simulink model "DLH_BDK_PD_momen_PP_r2014b"  (R2014b)
settings: Solver=ode3  SolverMode=SingleTasking  StartTime=0.0  StopTime=10  FixedStep=0.001  RelTol=1e-3
undefined symbols (not defined in the file): ADAMS_cwd, ADAMS_exec, ADAMS_host, ADAMS_init, ADAMS_inputs, ADAMS_outputs, ADAMS_prefix, ADAMS_static, ADAMS_sysdir
libraries: simulink x1
settings Model: CovMetricSettings=dwe  CovHtmlReporting=off  covSaveCumulativeToWorkspaceVar=off  CovSaveSingleToWorkspaceVar=off  CovExternalEMLEnable=on  CovSFcnEnable=on  Creator=MTA  LastModifiedBy=Administrator
settings DataIOCC: LimitDataPoints=off  SaveFormat=StructureWithTime
settings DebuggingCC: SolverPrmCheckMsg=none  FrameProcessingCompatibilityMsg=error  SFUnexpectedBacktrackingDiag=error  SFNoUnconditionalDefaultTransitionDiag=error
settings HardwareCC: ProdBitPerPointer=64  ProdLargestAtomicFloat=Float  ProdIntDivRoundTo=Zero  ProdEndianess=LittleEndian  ProdHWDeviceType=Specified
settings ModelReferenceCC: PropagateSignalLabelsOutOfModel=on
settings GRTTargetCC: TargetLangStandard=C99 (ISO)  GeneratePreprocessorConditionals=Use local settings

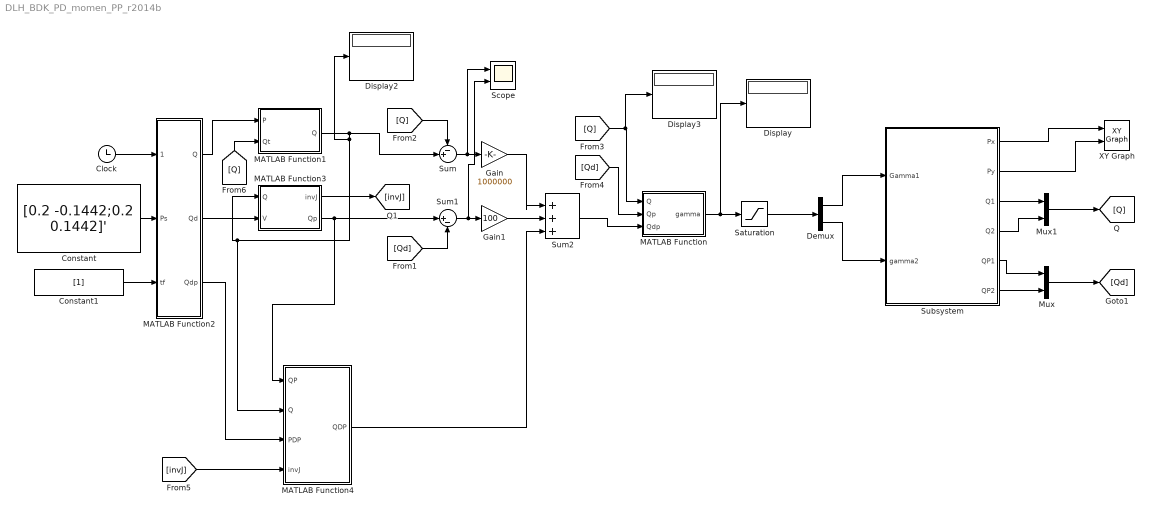
== system DLH_BDK_PD_momen_PP_r2014b ==
  Clock : Clock
  Constant : Constant  Value="[0.2  -0.1442;0.2 0.1442]'"
  Constant1 : Constant  Value=[1]
  Demux : Demux  Outputs=2
  Display : Display
  Display2 : Display
  Display3 : Display
  Gain : Gain  Gain=1000000
  Gain1 : Gain  Gain=100
  MATLAB Function : MATLAB Function  TreatAsAtomicUnit=on
      settings: PermitHierarchicalResolution=ParametersOnly
  MATLAB Function1 : MATLAB Function  TreatAsAtomicUnit=on
      settings: PermitHierarchicalResolution=ParametersOnly
  MATLAB Function2 : MATLAB Function  TreatAsAtomicUnit=on
      settings: PermitHierarchicalResolution=ParametersOnly
  MATLAB Function3 : MATLAB Function  TreatAsAtomicUnit=on
      settings: PermitHierarchicalResolution=ParametersOnly
  MATLAB Function4 : MATLAB Function  TreatAsAtomicUnit=on
      settings: PermitHierarchicalResolution=ParametersOnly
  Mux : Mux  Inputs=2
  Mux1 : Mux  Inputs=2
  Saturation : Saturate  UpperLimit=[5;5]  LowerLimit=[-5;-5]
  Scope : Scope  NumInputPorts=2
      settings: TimeRange=auto  MaxDataPoints=5000  SaveToWorkspace=off  SaveName=ScopeData  YMin=-469.58587~-5  YMax=523.49918~5  SampleTime=-1
  Subsystem : Subsystem
  Sum : Sum  Inputs=-+|
  Sum1 : Sum  Inputs=|+-
  Sum2 : Sum  Inputs=|+++
  XY Graph : simulink/Sinks/XY Graph  xmin=-1  xmax=1  ymin=-1  ymax=1  st=-1
  wires:
  Constant/1 -> MATLAB Function2/2(Ps)
  Constant1/1 -> MATLAB Function2/3(tf)
  Clock/1 -> MATLAB Function2/1(time)
  Sum/1 -> Scope/1, Gain/1
  Gain/1 -> Sum2/1
  Gain1/1 -> Sum2/2
  Sum1/1 -> Scope/2, Gain1/1
  Sum2/1 -> MATLAB Function/3(Qdp)
  Subsystem/2("Py ") -> XY Graph/2
  Subsystem/1("Px ") -> XY Graph/1
  Mux1/1 -> [Q]
  Mux/1 -> [Qd]
  Demux/2 -> Subsystem/2(gamma2)
  Subsystem/6(QP2) -> Mux/2
  Demux/1 -> Subsystem/1(Gamma1)
  Subsystem/4("Q2 ") -> Mux1/2
  Subsystem/3("Q1 ") -> Mux1/1
  Subsystem/5(QP1) -> Mux/1
  Saturation/1 -> Demux/1
  [Q] -> Sum/1
  [Qd] -> Sum1/2
  [Q] -> Display3/1, MATLAB Function/1(Q)
  MATLAB Function/1(gamma) -> Display/1, Saturation/1
  [Qd] -> MATLAB Function/2(Qp)
  MATLAB Function2/1(Q) -> MATLAB Function1/1(P)
  MATLAB Function1/1(Q) -> MATLAB Function4/2(Q), MATLAB Function3/1(Q), Display2/1, Sum/2
  MATLAB Function3/2(Qp) -> MATLAB Function4/1(QP), Sum1/1
  MATLAB Function2/2(Qd) -> MATLAB Function3/2(V)
  MATLAB Function2/3(Qdp) -> MATLAB Function4/3(PDP)
  MATLAB Function3/1(invJ) -> [invJ]
  [invJ] -> MATLAB Function4/4(invJ)
  MATLAB Function4/1(QDP) -> Sum2/3
  [Q] -> MATLAB Function1/2(Qt)

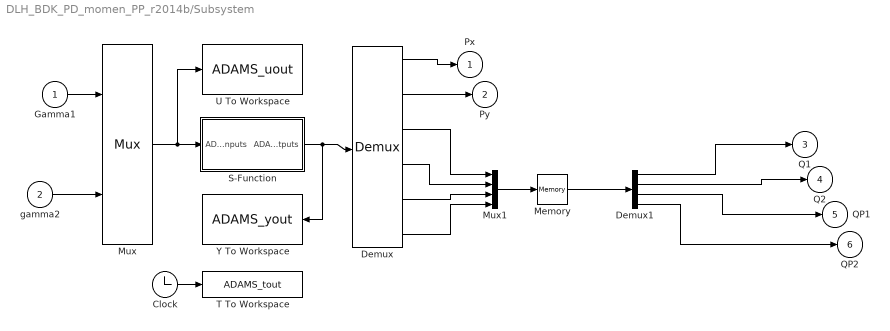
== system DLH_BDK_PD_momen_PP_r2014b/Subsystem ==
  Gamma1 : Inport
  gamma2 : Inport  Port=2
  Clock : Clock
  Demux : Demux  Outputs=6
  Demux1 : Demux
  Memory : Memory  X0=[0 ;-pi/2;0 ;0]
  Mux : Mux  Inputs=2
  Mux1 : Mux
  S-Function : Subsystem  LoadFcn=|  InitFcn=clear mex  mask(Adams Plant){exevie=ADAMS_sysdir, nam_in=ADAMS_inputs, namout=ADAMS_outputs, nampre=ADAMS_prefix, outfil=ADAMS_prefix, exesol=ADAMS_exec, stat=ADAMS_static, inicmd=[ADAMS_init], exetyp=C++, comtyp=PIPE(DDE), workdir=ADAMS_cwd, ada_host=ADAMS_host, modani=interactive, modsim=discrete, dft=no, simulink_lead_cosim=yes, pin_interp_order=0, pout_extrap_order=0, pin_extrap_order=0, pout_interp_order=0, dt_out=0.005, o_rate=1, more=off}
      | %check based on dialog box setting for when setting by popup menu                                             
      | if exist('ADAMS_solver_type')                                                                                 
      |   if strcmp(ADAMS_solver_type,'C++')                                                                          
      |     set_param(gcb,'exetyp','C++');                                                                            
      |   else                                                                                                        
      |     set_param(gcb,'exetyp','Fortran');                                                                        
      |   end                                                                                                         
      | else                                                                                                          
      |   set_param(gcb,'exetyp','C++');                                                                              
      | end                                                                                                           
      | %set the mode if using acar_solver                                                                            
      | %REQUIRED HERE BECAUSE BELOW CAUSES MDLTERMINATE TO BE CALLED 2 TIMES IN MIDDLE OF SIMULATION WHEN SET IN MASK
      |                                                                                                               
      | %enable the direct feedthrough, sim mode, anim mode parameters by default                                     
      |                                                                                                               
      | if exist('set_some_params_states')                                                                            
      |                                                                                                               
      |   set_some_params_states({'dft','modsim','modani'},{'on','on','on'},'MaskEnables',gcb)                        
      |   %turn on direct feedthrough option                                                                          
      |   set_some_params_states({'dft'},{'on'},'MaskVisibilities',gcb)                                               
      |                                                                                                               
      |  end                                                                                                          
      |                                                                                                               
      |                                                                                                               
      | if exist('ADAMS_exec')                                                                                        
      |   if and(strcmp(get_param(gcb,'exesol'),'ADAMS_exec'),strcmp(ADAMS_exec,'acar_solver'))                       
      |     %set the sim mode to discrete -- only supported mode                                                      
      |     set_param(gcb,'modsim','discrete')                                                                        
      |      %turn off direct feedthrough option                                                                      
      |      set_some_params_states({'dft'},{'off'},'MaskVisibilities',gcb)                                           
      |     %set the animation mode to batch -- only supported mode                                                   
      |     set_param(gcb,'modani','batch')                                                                           
      |     %disable the direct feedthrough, sim mode, anim mode parameters                                           
      |     set_some_params_states({'modsim','modani'},{'off','off'},'MaskEnables',gcb)                               
      |   end                                                                                                         
      | end
      mask prompts: exevie "Adams install directory"; nam_in "Adams View input names"; namout "Adams View output names"; nampre "Adams model file prefix"; outfil "Output files prefix (opt.: if blank - no output)"; exesol "User executable (opt.: if blank - use standard)"; stat "Initial static simulation flag"; inicmd "Initialization commands"; exetyp "Adams Solver type"; comtyp "Interprocess option"; workdir "Adams working directory"; ada_host "Adams host"; modani "Animation mode"; modsim "Simulation mode"; dft "Direct feedthrough"; simulink_lead_cosim "Discrete Computational Order - Simulink Leads Adams"; pin_interp_order "Plant input interpolation order"; pout_extrap_order "Plant output extrapolation order"; pin_extrap_order "Plant input extrapolation order"; pout_interp_order "Plant output interpolation order"; dt_out "Communication interval"; o_rate "Number of communications per output step"; more "More parameters"
      mask help: Simulate any Adams plant model either in Adams Solver form (.adm file) or in Adams View form (.cmd file)
      settings: OpenFcn=|
      | open_system(gcb,'mask')
      | if not(exist('set_some_params_states'))
      | 
      | warning('The script "set_some_params_states.m" cannot be found in the MATLAB PATH.  Cannot update the ADAMS Plant S-Function parameters.')
      | 
      | warning('Recommended action(optional):  run the Adams Controls .m file first to help choose the correct settings in the Adams S-Function block.')
      | 
      | end
      mask Help:
      | <html>
      | This S-Function represents the non-linear Adams Plant with the inputs sent to the Adams model <br>
      |  and the outputs generated by the Adams model.  See the Adams Controls documentation for more <br>
      | information.  This plant uses the following variables:<br>
      | <br>
      | <b>ADAMS_sysdir  :</b> Adams installation directory<br>
      | <b>ADAMS_inputs  :</b> Input variables View names vector<br>
      | <b>ADAMS_outputs :</b> Outputs variables View names vector<br>
      | <b>ADAMS_prefix  : </b>ADAMS model files prefix (.adm, .cmd); also doubles as output files prefix<br>
      | <b>ADAMS_exec :</b> Adams Solver user library or keyword (e.g., acar_solver)<br>
      | <b>ADAMS_static :</b> yes|no - initial static before Co-simulation(discrete)/Function Evaluation(continuous)<br>
      | <b>ADAMS_init :</b>Initialization commands (i.e., Adams View or Solver commands, depending on setting for Animation mode)<br>
      | <b>ADAMS_cwd : </b> Current working directory (for TCP/IP)<br>
      | <b>ADAMS_host : </b>Name of Adams server host (for TCP/IP)<br>
      | <b>ADAMS_mode :</b> Linear or non-linear (i.e., co-sim, function eval)<br>
      | <b>ADAMS_solver_type :</b>Fortran or C++ (used to set popup menu when first loaded) <br>
      | 
      | 
      | <br>
      | The following settings can be chosen:<br>
      | <br>
      | <b>Adams Solver type:</b>  Fortran or C++ (will also set ADAMS_solver_type)<br>
      | <b>Interprocess option:</b> Pipe(DDE) or TCP/IP; TCP/IP can allow different machines run Adams and MATLAB<br>
      | <b>Animation mode:</b> batch (Solver, uses .adm) or interactive (View, uses .cmd)<br>
      | <b>Simulation mode:</b> discrete (Co-simulation) or continuous (Function Evaluation)<br>
      | <b>Discrete Computational Order - Simulink Lead Adams:</b> for discrete mode, chooses if Simulink leads the integration (yes) or lags (no);<br> if set to "no", can remove algebraic loop<br>
      | <b>Plant input interpolation order:</b> 0 = zero-order hold; 1 = linear (discrete mode only, where Simulink leads)<br>
      | <b>Plant output extrapolation order:</b> 0 = zero-order hold;1 = linear(discrete mode only, where Simulink leads)<br>
      | <b>Plant input extrapolation order:</b> 0 = zero-order hold; 1 = linear (discrete mode only, where Adams leads)<br>
      | <b>Plant output interpolation order:</b> 0 = zero-order hold;1 = linear(discrete mode only, where Adams leads)<br>
      | <b>Direct feedthrough:</b> yes|no - yes = Input directly effect output(continuous mode-only)<br>
      | <b>Communication interval:</b> Time step at which Co-simulation exchange information (e.g.,0.005); also controls <br>output for continuous mode (Function Evaluation)<br>
      | <b>Number of communications per output step: </b>Sets Adams output rate (.res, .req, .gra) integer value (default: 1)<br>
      | </html>
      mask Callback exesol:
      | if exist('set_some_params_states')
      | %enable the direct feedthrough, sim mode, anim mode parameters
      | set_some_params_states({'dft','modsim','modani'},{'on','on','on'},'MaskEnables',gcb)
      | %turn on direct feedthrough option
      | set_some_params_states({'dft'},{'on'},'MaskVisibilities',gcb)
      | end
      | 
      | if exist('ADAMS_exec')
      |   if and(strcmp(get_param(gcb,'exesol'),'ADAMS_exec'),strcmp(ADAMS_exec,'acar_solver'))
      |     %set the sim mode to discrete -- only supported mode
      |     %REMOVED:  BELOW CAUSES MDLTERMINATE TO BE CALLED 2 TIMES IN MIDDLE OF SIMULATION
      |     %Now in LoadFcn callback
      |     %set_param(gcb,'modsim','discrete')
      |      %turn off direct feedthrough option
      |     set_some_params_states({'dft'},{'off'},'MaskVisibilities',gcb)
      |     %set the animation mode to batch -- only supported mode
      |     %REMOVED:  BELOW CAUSES MDLTERMINATE TO BE CALLED 2 TIMES IN MIDDLE OF SIMULATION
      |     %Now in LoadFcn callback
      |     %set_param(gcb,'modani','batch')
      |     %disable the direct feedthrough, sim mode, anim mode parameters
      |     set_some_params_states({'modsim','modani'},{'off','off'},'MaskEnables',gcb)
      |   end
      | end
      mask TypeOptions exetyp: Fortran | C++
      mask Callback exetyp:
      | if strcmp(get_param(gcb,'exetyp'),'C++')
      |     ADAMS_solver_type='C++';
      | else
      |     ADAMS_solver_type='Fortran';
      | end
      mask TypeOptions comtyp: PIPE(DDE) | TCP/IP
      mask Callback comtyp:
      | if exist('set_some_params_states')
      | if strcmp(get_param(gcb,'comtyp'),'PIPE(DDE)')
      |     %turn off cwd, host options
      |     set_some_params_states({'ada_host','workdir'},{'off','off'},'MaskVisibilities',gcb)
      | else%if strcmp(get_param(gcb,'modsim'),'TCP/IP')
      |     %turn on cwd, host options
      |     set_some_params_states({'ada_host','workdir'},{'on','on'},'MaskVisibilities',gcb)
      | end
      | end
      mask TypeOptions modani: batch | interactive
      mask TypeOptions modsim: discrete | continuous
      mask Callback modsim:
      | if exist('set_some_params_states')
      | if strcmp(get_param(gcb,'modsim'),'discrete')
      |      %turn off direct feedthrough option
      |     set_some_params_states({'dft'},{'off'},'MaskVisibilities',gcb)
      |     %turn on discrete co-sim type if want to see more
      |     if strcmp(get_param(gcb,'more'),'on')
      |         set_some_params_states({'simulink_lead_cosim'},{'on'},'MaskVisibilities',gcb)
      |     end
      |     if strcmp(get_param(gcb,'simulink_lead_cosim'),'yes')
      |         %turn on interpolation/extrapolation options
      |         set_some_params_states({'pin_interp_order','pout_extrap_order',},{'on','on'},'MaskVisibilities',gcb)
      |     else
      |         set_some_params_states({'pin_extrap_order','pout_interp_order'},{'on','on'},'MaskVisibilities',gcb)
      |     end
      | else%if strcmp(get_param(gcb,'modsim'),'continuous')
      |      %turn off direct feedthrough option
      |     set_some_params_states({'dft'},{'on'},'MaskVisibilities',gcb)
      |     %turn off interpolation/extrapolation options
      |     set_some_params_states({'pin_interp_order','pout_extrap_order','pin_extrap_order','pout_interp_order','simulink_lead_cosim'},{'off','off','off','off','off'},'MaskVisibilities',gcb)
      | end
      | end
      mask TypeOptions dft: no | yes
      mask TypeOptions simulink_lead_cosim: yes | no
      mask Callback simulink_lead_cosim:
      | if exist('set_some_params_states')
      | if (strcmp(get_param(gcb,'simulink_lead_cosim'),'yes') && strcmp(get_param(gcb,'modsim'),'discrete'))
      |      %turn off unused interpolate/extrapolate options
      |     set_some_params_states({'pin_extrap_order','pout_interp_order'},{'off','off'},'MaskVisibilities',gcb)
      |     %turn on used interpolate/extrapolate options
      |     set_some_params_states({'pin_interp_order','pout_extrap_order'},{'on','on'},'MaskVisibilities',gcb)
      | elseif (strcmp(get_param(gcb,'simulink_lead_cosim'),'no') && strcmp(get_param(gcb,'modsim'),'discrete'))
      |     %turn on used interpolate/extrapolate options
      |     set_some_params_states({'pin_extrap_order','pout_interp_order'},{'on','on'},'MaskVisibilities',gcb)
      |      %turn off unused interpolate/extrapolate options
      |     set_some_params_states({'pin_interp_order','pout_extrap_order'},{'off','off'},'MaskVisibilities',gcb)
      | end
      | end
      mask TypeOptions pin_interp_order: 0 | 1
      mask TypeOptions pout_extrap_order: 0 | 1
      mask TypeOptions pin_extrap_order: 0 | 1
      mask TypeOptions pout_interp_order: 0 | 1
      mask Callback more:
      | if exist('set_some_params_states')
      | if (strcmp(get_param(gcb,'more'),'on'))
      |      %turn on infrequently used options
      |     set_some_params_states({'exevie','nam_in','namout','exesol','stat','inicmd'},{'on','on','on','on','on','on'},'MaskVisibilities',gcb)
      |     if strcmp(get_param(gcb,'modsim'),'discrete')
      |         set_some_params_states({'simulink_lead_cosim'},{'on'},'MaskVisibilities',gcb)
      |     end
      | elseif (strcmp(get_param(gcb,'more'),'off'))
      |     %turn off infrequently used options
      |     set_some_params_states({'exevie','nam_in','namout','exesol','stat','inicmd'},{'off','off','off','off','off','off'},'MaskVisibilities',gcb)
      |     if strcmp(get_param(gcb,'modsim'),'discrete')
      |         set_some_params_states({'simulink_lead_cosim'},{'off'},'MaskVisibilities',gcb)
      |     end
      | end
      | end
      mask Display: disp( 'MSC Software' )
  T To Workspace : ToWorkspace  VariableName=ADAMS_tout
      settings: MaxDataPoints=100000
  U To Workspace : ToWorkspace  VariableName=ADAMS_uout
      settings: MaxDataPoints=100000
  Y To Workspace : ToWorkspace  VariableName=ADAMS_yout
      settings: MaxDataPoints=100000
  "Px " : Outport
  "Py " : Outport  Port=2
  "Q1 " : Outport  Port=3
  "Q2 " : Outport  Port=4
  QP1 : Outport  Port=5
  QP2 : Outport  Port=6
  wires:
  Demux/1 -> "Px "/1
  Demux/2 -> "Py "/1
  Demux1/2 -> "Q2 "/1
  Demux/3 -> Mux1/1
  Demux/4 -> Mux1/2
  Demux/5 -> Mux1/3
  Demux/6 -> Mux1/4
  Mux1/1 -> Memory/1
  Memory/1 -> Demux1/1
  Demux1/1 -> "Q1 "/1
  Demux1/3 -> QP1/1
  Demux1/4 -> QP2/1
  gamma2/1 -> Mux/2
  Clock/1 -> T To Workspace/1
  Gamma1/1 -> Mux/1
  S-Function/1(ADAMS outputs) -> Demux/1, Y To Workspace/1
  Mux/1 -> S-Function/1(ADAMS inputs), U To Workspace/1

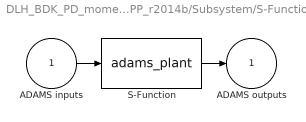
== system DLH_BDK_PD_momen_PP_r2014b/Subsystem/S-Function ==
  ADAMS inputs : Inport
  S-Function : S-Function  StopFcn=clear mex  FunctionName=adams_plant  Parameters=exevie,exesol,stat,outfil,nampre,o_rate,nam_in,namout,dft,modsim,modani,dt_out,inicmd,exetyp,comtyp,ada_host, workdir,pin_interp_order,pout_extrap_order,pin_extrap_order,pout_interp_order,simulink_lead_cosim  SFunctionDeploymentMode=off  EnableBusSupport=off
  ADAMS outputs : Outport  InitialOutput=0
  wires:
  S-Function/1 -> ADAMS outputs/1
  ADAMS inputs/1 -> S-Function/1

== matlab function DLH_BDK_PD_momen_PP_r2014b/MATLAB Function1 ==
  data: P input; Q output; Qt input
function Q = IGM(P,Qt)
L1=0.2;
L2=0.1442;
x=P(1);
y=P(2);
q2=-acos((x^2+y^2-L1^2-L2^2)/2/L1/L2);
q1=cmp(x,y,L1,L2,q2);
k=1;
while ((q1<0)&&(Qt(1)>(2*k-1)*pi/2))
    q1=q1+2*k*pi;
    k=k+1;
end
k=1;
while ((q1>=0)&&(Qt(1)>(2*k+1)*pi/2)&&(q1<=pi))
    q1=q1+2*k*pi;
    k=k+1;
end
Q=[q1;q2];
function q1=cmp(x,y,L1,L2,q2)
L1x=L1+L2*cos(q2);
L1y=L2*sin(q2);
q=[L1x -L1y;L1y L1x]\[x;y];
q1=atan2(q(2),q(1));

== matlab function DLH_BDK_PD_momen_PP_r2014b/MATLAB Function ==
  data: Q input; gamma output; Qp input; Qdp input
function gamma = IDM(Q,Qp,Qdp)
gamma=zeros(2,1);
Q2=Q(2);
Qp1=Qp(1);
Qp2=Qp(2);
Qdp1=Qdp(1);
Qdp2=Qdp(2);
M1 = 1.4899
L1=0.2;M2=0.464;ZZ1=0.0045;ZZ2=0.00156;
MY2=0;MX2=0.025686;
gamma(1) = Qdp1*(ZZ1 + ZZ2 + L1^2*M2 + 2*L1*MX2*cos(Q2) - 2*L1*MY2*sin(Q2)) + Qdp2*(ZZ2 + L1*MX2*cos(Q2) - L1*MY2*sin(Q2)) - L1*Qp2*(Qp1 + Qp2)*(MY2*cos(Q2) + MX2*sin(Q2)) - L1*Qp1*Qp2*(MY2*cos(Q2) + MX2*sin(Q2));
gamma(2) =  Qdp2*ZZ2 + Qdp1*(ZZ2 + L1*MX2*cos(Q2) - L1*MY2*sin(Q2)) + (L1*Qp1*(MY2*cos(Q2) + MX2*sin(Q2))*(Qp1 - Qp2))/2;
 end

== matlab function DLH_BDK_PD_momen_PP_r2014b/MATLAB Function2 ==
  data: time input; Ps input; tf input; Q output; Qd output; Qdp output
function [Q,Qd,Qdp] = fcn(time,Ps,tf)
n=length(tf);
[k,tk_1] = find(time,tf,n);
if(k==1)
    t=min(time/tf(1),1);
else
    t = min((time-tk_1)/tf(k),1);
end
r=10*t^3-15*t^4+6*t^5;
rd=30*t^2-60*t^3+30*t^4;
r2d=60*t-180*t^2+120*t^3;
D=Ps(:,k+1)-Ps(:,k);
Q=Ps(:,k)+r*D;
Qd=rd*D;
Qdp=r2d*D;
function [k,tk_1]=find(time,tf,n)
t=0;
k=n;
for i=1:n
    tk=t+tf(i);
    if(t<=time)&&(time<tk)
        k=i;
        break;
    end
    t=tk;
    if(i==n)
        t=tk-tf(n);
    end
end
tk_1=t;

== matlab function DLH_BDK_PD_momen_PP_r2014b/MATLAB Function3 ==
  data: Q input; invJ output; V input; Qp output
function [invJ,Qp] = IDM(Q,V)
L1=0.2;
L2=0.1442;
q1=Q(1);
q2=Q(2);
c1=cos(q1);
s1=sin(q1);
c12=cos(q1+q2);
s12=sin(q1+q2);
J=[-L2*s12-L1*s1,-L2*s12;
    L2*c12+L1*c1,L2*c12];
Qp=J^-1*V;
invJ=J^-1;

== matlab function DLH_BDK_PD_momen_PP_r2014b/MATLAB Function4 ==
  data: QP input; QDP output; Q input; PDP input; invJ input
function QDP  = HHH(QP,Q,PDP,invJ)
L1=0.2;
L2=0.1442;
q1=Q(1);
q2=Q(2);
c1=cos(q1);
s1=sin(q1);
c12=cos(q1+q2);
s12=sin(q1+q2);
Jp=[-L2*c12*(QP(1)+QP(2))-L1*c1*QP(1), -L2*c12*(QP(1)+QP(2))
    -L2*s12*(QP(1)+QP(2))-L1*s1*QP(1), -L2*s12*(QP(1)+QP(2))];
QDP=invJ*(PDP-Jp*QP);
